simulink model "ballsegway_model"  (R2024b)
settings: Solver=VariableStepAuto  StartTime=0.0  StopTime=10  RelTol=1e-3
libraries: simulink x2
settings Model: Creator=sumit  LastModifiedBy=yugan
settings DebuggingCC: AlgebraicLoopMsg=none

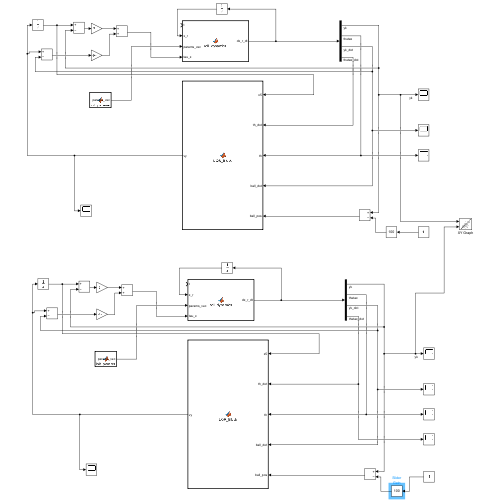
[thumbnail: Simulink's stored preview of the top-level diagram]
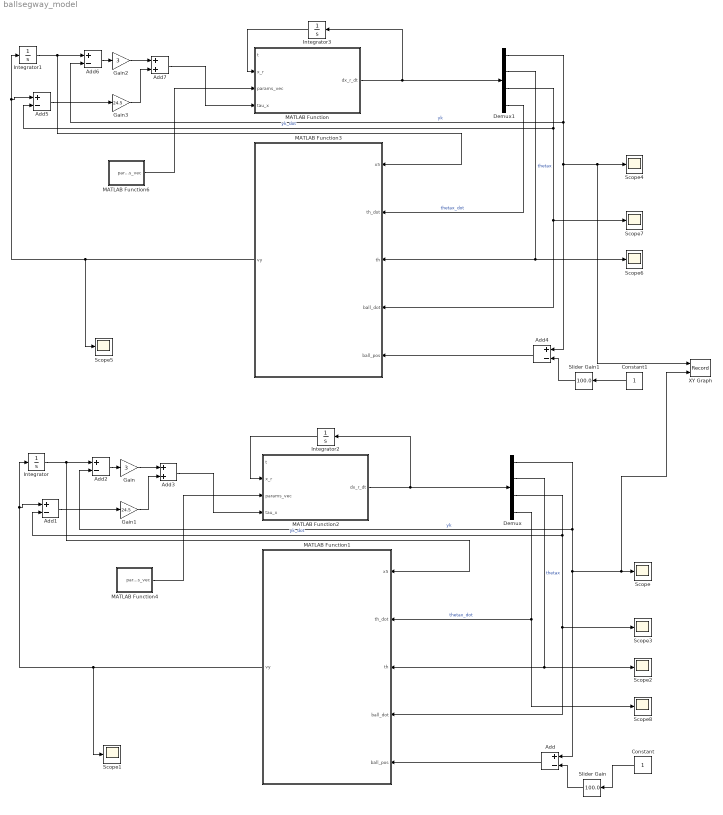
== system ballsegway_model ==
  Add{,1..2,4..6} (6 alike) : Sum  Inputs=+-
  Add3 : Sum
  Add7 : Sum
  Constant : Constant
  Constant1 : Constant
  Demux : Demux
  Demux1 : Demux
  Gain : Gain  Gain=3
  Gain1 : Gain  Gain=24.5
  Gain2 : Gain  Gain=3
  Gain3 : Gain  Gain=24.5
  Integrator : Integrator
  Integrator1 : Integrator
  Integrator2 : Integrator  InitialCondition=[0; 0; 0; 0]
  Integrator3 : Integrator  InitialCondition=[0; 0; 0; 0]
  MATLAB Function : MATLAB Function  TreatAsAtomicUnit=on
  MATLAB Function1 : MATLAB Function  TreatAsAtomicUnit=on
  MATLAB Function2 : MATLAB Function  TreatAsAtomicUnit=on
  MATLAB Function3 : MATLAB Function  TreatAsAtomicUnit=on
  MATLAB Function4 : MATLAB Function  TreatAsAtomicUnit=on
  MATLAB Function6 : MATLAB Function  TreatAsAtomicUnit=on
  Scope{,1..8} (9 alike) : Scope
  Slider Gain : simulink/Math Operations/Slider Gain  gain=100.0  low=0  high=100
  Slider Gain1 : simulink/Math Operations/Slider Gain  gain=100.0  low=0  high=100
  XY Graph : Record  FileSettingsInternal="{\"entries\":[{\"content\":{\"excelSettings\":{\"content\":{},\"type\":\"Streamout.ExcelSettings\"}},\"type\":\"Streamout.FileSettingStorage\",\"uuid\":\"\"}],\"packageUris\":[\"http:\\/\\/schema.mathworks.com\\/mf0\\/streamout_blocks\\/R2020a\"],\"version\":\"1.0\"}"  Layout=[1 1]  SignalsInternal="{\"entries\":[{\"content\":{\"signals\":[{\"content\":{\"blockPath\":[],\"dimensions\":[1,1],\"domain\":\"\",\"lineColor\":\"#a2142f\",\"plots\":[ 1 ],\"port\":1,\"sid\":[\"\"],\"signalID\":1,\"signalName\":\"xk\"},\"type\":\"RecordBlkView.Signal\",\"uuid\":\"\"},{\"content\":{\"blockPath\":[],\"dimensions\":[1,1],\"domain\":\"\",\"lineColor\":\"#139fff\",\"plots\":[ 1 ],\"port\":2,\"sid\":[\"\"],\"signalID\":2,\"signalName\":\"yk\"},\"type\":\"RecordBlkView.Signal\",\"uuid\":\"\"}]},\"type\":\"RecordBlkView.InputSignals\",\"uuid\":\"\"}],\"packageUris\":[\"http:\\/\\/schema.mathworks.com\\/mf0\\/streamout_blocks\\/R2020a\"],\"version\":\"1.0\"}"  VisualizationBindings="{\"xyplotplugin\":{\"info\":[{\"series\":[{\"bindingParametersList\":[{\"parameter\":\"X-Axis\",\"signalID\":1,\"signalName\":\"yk\"},{\"parameter\":\"Y-Axis\",\"signalID\":2,\"signalName\":\"yk\"}],\"seriesID\":0}],\"subplotID\":1}]}}"  CompatibilityTag=XY
  wires:
  Integrator2/1 -> MATLAB Function2/2(x_r)
  MATLAB Function2/1(dx_r_dt) -> Integrator2/1, Demux/1
  Demux/1 -> Add/1, XY Graph/2, Scope/1, Add2/2  "yk"
  Add/1 -> MATLAB Function1/5(ball_pos)
  Constant/1 -> Slider Gain/1
  Demux/2 -> Scope2/1, MATLAB Function1/3(th)  "thetax"
  Demux/3 -> MATLAB Function1/4(ball_dot), Scope3/1, Add1/2  "yk_dot"
  Demux/4 -> Scope8/1, MATLAB Function1/2(th_dot)  "thetax_dot"
  MATLAB Function1/1(vy) -> Scope1/1, Add1/1, Integrator/1
  Integrator/1 -> MATLAB Function1/1(x5), Add2/1
  Add2/1 -> Gain/1
  Gain/1 -> Add3/1
  Add3/1 -> MATLAB Function2/4(tau_x)
  MATLAB Function4/1(params_vec) -> MATLAB Function2/3(params_vec)
  Add1/1 -> Gain1/1
  Gain1/1 -> Add3/2
  Slider Gain/1 -> Add/2
  Add7/1 -> MATLAB Function/4(tau_x)
  MATLAB Function6/1(params_vec) -> MATLAB Function/3(params_vec)
  MATLAB Function3/1(vy) -> Scope5/1, Add5/1, Integrator1/1
  Demux1/3 -> MATLAB Function3/4(ball_dot), Scope7/1, Add5/2  "yk_dot"
  Gain2/1 -> Add7/1
  Add5/1 -> Gain3/1
  Integrator1/1 -> MATLAB Function3/1(x5), Add6/1
  Integrator3/1 -> MATLAB Function/2(x_r)
  MATLAB Function/1(dx_r_dt) -> Integrator3/1, Demux1/1
  Demux1/1 -> Add4/1, XY Graph/1, Scope4/1, Add6/2  "yk"
  Add6/1 -> Gain2/1
  Slider Gain1/1 -> Add4/2
  Constant1/1 -> Slider Gain1/1
  Demux1/4 -> MATLAB Function3/2(th_dot)  "thetax_dot"
  Demux1/2 -> Scope6/1, MATLAB Function3/3(th)  "thetax"
  Add4/1 -> MATLAB Function3/5(ball_pos)
  Gain3/1 -> Add7/2

== matlab function ballsegway_model/MATLAB Function3 ==
  data: x5 input; th_dot input; th input; ball_dot input; ball_pos input; vy output size=[1]
function vy  = LQR_Block(x5, th_dot, th, ball_dot, ball_pos)
%(x5, th, th_dot, )
% ========================================================================
%   REAL-TIME LQR CONTROLLER BLOCK
%   Applies pre-calculated gains Kr and Kp to the system states.
%
%   This block EXPECTS 'Kr' and 'Kp' to be passed in as parameters.
% ========================================================================

%% ------------------------------------------------------------
% BUILD STATE VECTORS
% **FIXED**: Swapped states back. Roll (y/2) and Pitch (x/1)
%            Please verify th(1) vs th(2) matches your setup.
%            Commonly: th(1)=pitch, th(2)=roll
%% ------------------------------------------------------------

Kr = [0.98, 7.45, 9.88, 0.09, 0];  % example row
  % example row


xr = [ th;         % Roll angle
       th_dot;     % Roll rate
       ball_pos;   % Ball X position (relative to roll)
       ball_dot;   % Ball X velocity
       x5          % Roll integral term
       ];
       


%% ------------------------------------------------------------
% CONTROL LAWS (Simple multiplication)
%% ------------------------------------------------------------
vy = -Kr * xr;   % Roll command
   % Pitch command
end

== matlab function ballsegway_model/MATLAB Function2 ==
  data: t input; dx_r_dt output; x_r input; params_vec input; tau_x input
function dx_r_dt = roll_dynamics(t, x_r, params_vec, tau_x)
% roll_dynamics.m
%
% State vector x_r = [y_k, theta_x, y_k_dot, theta_x_dot]'

%% 1. Unpack State
y_k         = x_r(1);
theta_x     = x_r(2);
y_k_dot     = x_r(3);
theta_x_dot = x_r(4);
q_x_dot     = [y_k_dot; theta_x_dot];

%% 2. Unpack parameters from vector
mk  = params_vec(1);
Ik  = params_vec(2);
ma  = params_vec(3);
Ix  = params_vec(4);
Iy  = params_vec(5);
Iz  = params_vec(6);
l   = params_vec(7);
alpha_rad = params_vec(8);
rk  = params_vec(9);
rw  = params_vec(10);
bx  = params_vec(11);
dx  = params_vec(12);
by  = params_vec(13);   % USED
dy  = params_vec(14);   % USED
bry = params_vec(15);
dry = params_vec(16);
brx = params_vec(17);   % USED
drx = params_vec(18);   % USED
g   = params_vec(19);
k_motor = params_vec(20);

%% 3. Dynamics Matrices

% Mass Matrix
M11 = mk + (Ik / rk^2) + ma + (3*Iy*cos(alpha_rad)^2)/(2*rw^2);
M12 = (3*Iy*cos(alpha_rad)^2)/(2*rw^2)*rk - ma*l*cos(theta_x);
M21 = M12;
M22 = ma*l^2 + (3*Iy*rk^2*cos(alpha_rad)^2)/(2*rw^2) + Ix;
M_x = [M11 M12; M21 M22];

% Coriolis Matrix
C_x = [ 0                     ma*l*theta_x_dot*sin(theta_x);
        0                     0 ];

% Gravity Vector
G_x = [ 0 ;
       -ma*g*l*sin(theta_x) ];

%% 4. Friction / Damping Vector (NEW)
% D(q̇) = [by*y_k_dot + dy*sign(y_k_dot) ;
%         brx*theta_x_dot + drx*sign(theta_x_dot)]

D1 = by * y_k_dot     + dy  * sign(y_k_dot);
D2 = brx * theta_x_dot + drx * sign(theta_x_dot);
D_x = [D1 ; D2];

%% 5. Control torque vector
Q_x = [ (1/rw)*tau_x ;
         (rk/rw)*tau_x ];

%% 6. Compute accelerations
q_x_ddot = M_x \ (Q_x - C_x*q_x_dot - D_x - G_x);

%% 7. Output derivative
dx_r_dt = [
    y_k_dot ;
    theta_x_dot ;
    q_x_ddot(1) ;
    q_x_ddot(2)
];

end

== matlab function ballsegway_model/MATLAB Function6 ==
  data: params_vec output size=[20 1]
function params_vec = init_params()
% init_params.m
% Returns parameters as a 20×1 vector (NO STRUCT)

mk  = 19.6;                   % (1) ball mass
Ik  = 0.38;                   % (2) ball inertia
ma  = 68;                     % (3) body mass
Ix  = 12.1;                   % (4) body inertia x
Iy  = 11.67;                  % (5) body inertia y
Iz  = 1.08;                   % (6) body inertia z
l   = 0.38;                   % (7) COM height
a   = deg2rad(65.5);          % (8) zenith angle
rk  = 0.22;                   % (9) ball radius
rw  = 0.10;                   % (10) omniwheel radius
bx  = 0.10;                   % (11) viscous friction xz
dx  = 0.01;                   % (12) coulomb friction xz
by  = 0.10;                   % (13) viscous friction yz
dy  = 0.01;                   % (14) coulomb friction yz
bry = 0.12;                   % (15) body/ball viscous xz
dry = 0.02;                   % (16) coulomb xz
brx = 0.12;                   % (17) body/ball viscous yz
drx = 0.02;                   % (18) coulomb yz
g   = 9.81;                   % (19) gravity
k_motor = 1;                  % (20) motor constant


% Return as vector
params_vec = [
    mk; Ik; ma; Ix; Iy; Iz;
    l; a; rk; rw;
    bx; dx; by; dy;
    bry; dry; brx; drx;
    g; k_motor
];
end

== matlab function ballsegway_model/MATLAB Function4 ==
  data: params_vec output size=[20 1]
function params_vec = init_params()
% init_params.m
% Returns parameters as a 20×1 vector (NO STRUCT)

mk  = 19.6;                   % (1) ball mass
Ik  = 0.38;                   % (2) ball inertia
ma  = 68;                     % (3) body mass
Ix  = 12.1;                   % (4) body inertia x
Iy  = 11.67;                  % (5) body inertia y
Iz  = 1.08;                   % (6) body inertia z
l   = 0.38;                   % (7) COM height
a   = deg2rad(65.5);          % (8) zenith angle
rk  = 0.22;                   % (9) ball radius
rw  = 0.10;                   % (10) omniwheel radius
bx  = 0.10;                   % (11) viscous friction xz
dx  = 0.01;                   % (12) coulomb friction xz
by  = 0.10;                   % (13) viscous friction yz
dy  = 0.01;                   % (14) coulomb friction yz
bry = 0.12;                   % (15) body/ball viscous xz
dry = 0.02;                   % (16) coulomb xz
brx = 0.12;                   % (17) body/ball viscous yz
drx = 0.02;                   % (18) coulomb yz
g   = 9.81;                   % (19) gravity
k_motor = 1;                  % (20) motor constant


% Return as vector
params_vec = [
    mk; Ik; ma; Ix; Iy; Iz;
    l; a; rk; rw;
    bx; dx; by; dy;
    bry; dry; brx; drx;
    g; k_motor
];
end

== matlab function ballsegway_model/MATLAB Function ==
  data: t input; dx_r_dt output; x_r input; params_vec input; tau_x input
function dx_r_dt = roll_dynamics(t, x_r, params_vec, tau_x)
% roll_dynamics.m
%
% State vector x_r = [y_k, theta_x, y_k_dot, theta_x_dot]'

%% 1. Unpack State
y_k         = x_r(1);
theta_x     = x_r(2);
y_k_dot     = x_r(3);
theta_x_dot = x_r(4);
q_x_dot     = [y_k_dot; theta_x_dot];

%% 2. Unpack parameters from vector
mk  = params_vec(1);
Ik  = params_vec(2);
ma  = params_vec(3);
Ix  = params_vec(4);
Iy  = params_vec(5);
Iz  = params_vec(6);
l   = params_vec(7);
alpha_rad = params_vec(8);
rk  = params_vec(9);
rw  = params_vec(10);
bx  = params_vec(11);
dx  = params_vec(12);
by  = params_vec(13);   % USED
dy  = params_vec(14);   % USED
bry = params_vec(15);
dry = params_vec(16);
brx = params_vec(17);   % USED
drx = params_vec(18);   % USED
g   = params_vec(19);
k_motor = params_vec(20);

%% 3. Dynamics Matrices

% Mass Matrix
M11 = mk + (Ik / rk^2) + ma + (3*Iy*cos(alpha_rad)^2)/(2*rw^2);
M12 = (3*Iy*cos(alpha_rad)^2)/(2*rw^2)*rk - ma*l*cos(theta_x);
M21 = M12;
M22 = ma*l^2 + (3*Iy*rk^2*cos(alpha_rad)^2)/(2*rw^2) + Ix;
M_x = [M11 M12; M21 M22];

% Coriolis Matrix
C_x = [ 0                     ma*l*theta_x_dot*sin(theta_x);
        0                     0 ];

% Gravity Vector
G_x = [ 0 ;
       -ma*g*l*sin(theta_x) ];

%% 4. Friction / Damping Vector (NEW)
% D(q̇) = [by*y_k_dot + dy*sign(y_k_dot) ;
%         brx*theta_x_dot + drx*sign(theta_x_dot)]

D1 = by * y_k_dot     + dy  * sign(y_k_dot);
D2 = brx * theta_x_dot + drx * sign(theta_x_dot);
D_x = [D1 ; D2];

%% 5. Control torque vector
Q_x = [ (1/rw)*tau_x ;
         (rk/rw)*tau_x ];

%% 6. Compute accelerations
q_x_ddot = M_x \ (Q_x - C_x*q_x_dot - D_x - G_x);

%% 7. Output derivative
dx_r_dt = [
    y_k_dot ;
    theta_x_dot ;
    q_x_ddot(1) ;
    q_x_ddot(2)
];

end

== matlab function ballsegway_model/MATLAB Function1 ==
  data: x5 input; th_dot input; th input; ball_dot input; ball_pos input; vy output size=[1]
function vy  = LQR_Block(x5, th_dot, th, ball_dot, ball_pos)
%(x5, th, th_dot, )
% ========================================================================
%   REAL-TIME LQR CONTROLLER BLOCK
%   Applies pre-calculated gains Kr and Kp to the system states.
%
%   This block EXPECTS 'Kr' and 'Kp' to be passed in as parameters.
% ========================================================================

%% ------------------------------------------------------------
% BUILD STATE VECTORS
% **FIXED**: Swapped states back. Roll (y/2) and Pitch (x/1)
%            Please verify th(1) vs th(2) matches your setup.
%            Commonly: th(1)=pitch, th(2)=roll
%% ------------------------------------------------------------

Kr = [0.98, 7.45, 9.88, 0.09, 0];  % example row
  % example row


xr = [ th;         % Roll angle
       th_dot;     % Roll rate
       ball_pos;   % Ball X position (relative to roll)
       ball_dot;   % Ball X velocity
       x5          % Roll integral term
       ];
       


%% ------------------------------------------------------------
% CONTROL LAWS (Simple multiplication)
%% ------------------------------------------------------------
vy = -Kr * xr;   % Roll command
   % Pitch command
end
